simulink model "PPC_P1"  (R2019b)
settings: Solver=ode45  StartTime=0.0  StopTime=50  MaxStep=0.01  RelTol=1e-6
undefined symbols (not defined in the file or in its folder): sigbuilder_block
libraries: slctrlblks x2, simulink x1
settings Model: Creator=Kevin  LastModifiedBy=Kevin

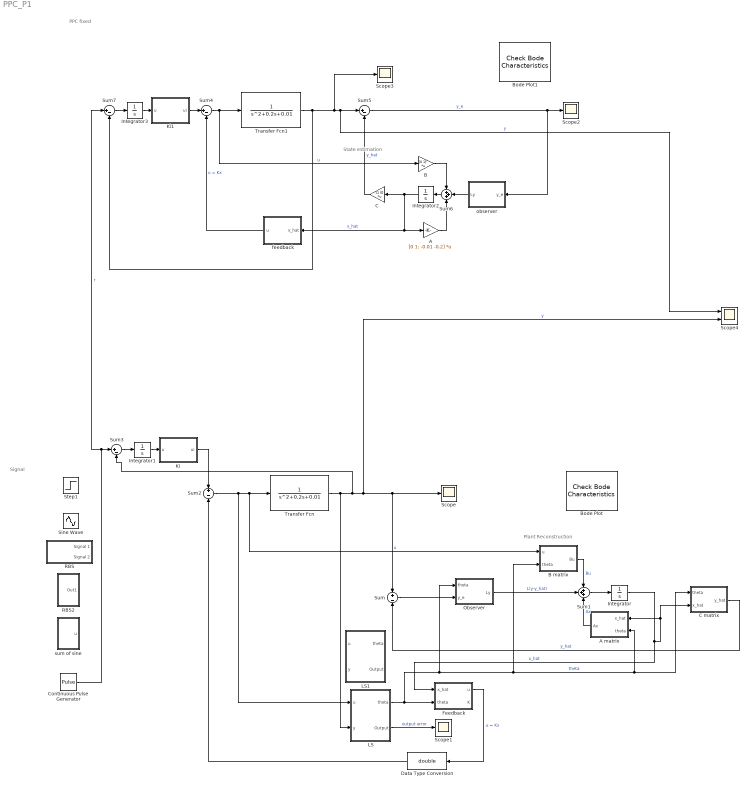
== system PPC_P1 ==
  note: PPC fixed
  note: Plant Reconstruction
  note: Signal
  note: State estimation
  A : Gain  Gain=[0 1; -0.01 -0.2]  Multiplication=Matrix(K*u)
  A matrix : MATLAB Function  TreatAsAtomicUnit=on
  B : Gain  Gain=[0 1]'  Multiplication=Matrix(K*u)
  B matrix : MATLAB Function  TreatAsAtomicUnit=on
  Bode Plot : slctrlblks/Model Verification/Check Bode  Characteristics  InstantiateOnLoad=on  SaveOperatingPoints=off  LinearizationIOs={'/Sum2', 1, 'in', 'off', '';'/Transfer Fcn', 1, 'out', 'on', ''}  LinearizeAt=SnapshotTimes  SnapshotTimes=[0]  TriggerType=rising  SampleTime=auto  RateConversionMethod=zoh  PreWarpFreq=10  UseExactDelayModel=off  UseFullBlockNameLabels=off  UseBusSignalLabels=off  enabled=on  stopWhenAssertionFail=off  export=off  ViewDlgPos=[1921 -319 1920 967.333333333333]  OpenViewOnLoad=off  LaunchViewOnOpen=off  FrequencyUnits=rad/s  MagnitudeUnits=dB  PhaseUnits=deg  TimeUnits=seconds  EnableUpperBound=off  UpperBoundFrequencies=[]  UpperBoundMagnitudes=[]  EnableLowerBound=off  LowerBoundFrequencies=[]  LowerBoundMagnitudes=[]
      settings: SourceProductName=Simulink Control Design
  Bode Plot1 : slctrlblks/Model Verification/Check Bode  Characteristics  InstantiateOnLoad=on  SaveOperatingPoints=off  LinearizationIOs={'/Sum', 1, 'in', 'off', '';'/Transfer Fcn', 1, 'out', 'on', ''}  LinearizeAt=SnapshotTimes  SnapshotTimes=[0]  TriggerType=rising  SampleTime=auto  RateConversionMethod=zoh  PreWarpFreq=10  UseExactDelayModel=off  UseFullBlockNameLabels=off  UseBusSignalLabels=off  enabled=on  stopWhenAssertionFail=off  export=off  ViewDlgPos=[1921 -319 1920 967.333333333333]  OpenViewOnLoad=off  LaunchViewOnOpen=off  FrequencyUnits=rad/s  MagnitudeUnits=dB  PhaseUnits=deg  TimeUnits=seconds  EnableUpperBound=off  UpperBoundFrequencies=[]  UpperBoundMagnitudes=[]  EnableLowerBound=off  LowerBoundFrequencies=[]  LowerBoundMagnitudes=[]
      settings: SourceProductName=Simulink Control Design
  C : Gain  Gain=[1 0]  Multiplication=Matrix(K*u)
  C matrix : MATLAB Function  TreatAsAtomicUnit=on
  Continuous Pulse Generator : DiscretePulseGenerator  PulseType=Time based  Period=1  PulseWidth=50
  Data Type Conversion : DataTypeConversion  OutDataTypeStr=double
  Feedback : MATLAB Function  TreatAsAtomicUnit=on
  Integrator{,1..3} (4 alike) : Integrator
  Ki : MATLAB Function  TreatAsAtomicUnit=on
  Ki1 : MATLAB Function  TreatAsAtomicUnit=on
  LS : Subsystem
  LS1 : Subsystem
  "Observer " : MATLAB Function  TreatAsAtomicUnit=on
  "RBS " : Subsystem  Tag=STV Subsys  LoadFcn=sigbuilder_block('load');  StartFcn=sigbuilder_block('start');  StopFcn=sigbuilder_block('stop');  ClipboardFcn=sigbuilder_block('clipboard');  mask(Sigbuilder block){tuvar=[0:10]}
      mask help: Simulink:masks:SigbuilderBlock_MD
      mask init:
      | if ~strcmp(get_param(bdroot(gcbh),'SimulationStatus'),'stopped') tuvar = sigbuilder_block('maskInit'); end
      settings: CopyFcn=sigbuilder_block('copy');  DeleteFcn=sigbuilder_block('delete');  ModelCloseFcn=sigbuilder_block('modelClose');  PreSaveFcn=sigbuilder_block('preSave');  PauseFcn=sigbuilder_block('pause');  ContinueFcn=sigbuilder_block('continue');  NameChangeFcn=sigbuilder_block('namechange');  OpenFcn=sigbuilder_block('open',[215 62.5 550.5 362.5 ]);  CloseFcn=sigbuilder_block('close');
      mask Display: plot(0, 0, 100, 100,[2, 2, 32, 32, 2], [68, 8, 8, 68, 68],[32, 2], [38, 38], [32, 19, 2],[53, 60, 44], [32, 17, 17, 2],[16, 16, 31, 31]);txt = getActiveGroup(gcbh);text(2, 100, txt,'verticalAlignment', 'top');
  RBS2 : Subsystem
  Scope{,1..3} (4 alike) : Scope
  Scope4 : Scope  NumInputPorts=2
  Sine Wave : Sin  Frequency=0.1  SampleTime=0
  Step1 : Step  SampleTime=0
  Sum : Sum  Inputs=+-
  Sum1 : Sum  Inputs=+++
  Sum2 : Sum  Inputs=+-
  Sum{3..5,7} (4 alike) : Sum  Inputs=|+-
  Sum6 : Sum  Inputs=+++
  Transfer Fcn : TransferFcn  Denominator=[1 ,0.2 ,0.01]
  Transfer Fcn1 : TransferFcn  Denominator=[1 ,0.2 ,0.01]
  feedback : MATLAB Function  TreatAsAtomicUnit=on
  "observer " : MATLAB Function  TreatAsAtomicUnit=on
  sum of sine : Subsystem
  wires:
  Transfer Fcn/1 -> LS/2(y), Sum3/2, Scope4/2, Scope/1, Sum/1  "y"
  Sum2/1 -> LS/1("u "), B matrix/1(u), Transfer Fcn/1  "u"
  LS/1(theta) -> C matrix/1(theta), A matrix/2(theta), B matrix/2(theta), "Observer "/1(theta), Feedback/2(theta)  "theta"
  Sum/1 -> "Observer "/2(y_e)
  Sum1/1 -> Integrator/1
  Integrator/1 -> C matrix/2(x_hat), A matrix/1(x_hat), Feedback/1(x_hat)  "x_hat"
  A matrix/1(Ax) -> Sum1/3  "Ax"
  "Observer "/1(Ly) -> Sum1/2  "L(y-y_hat)"
  C matrix/1(y_hat) -> Sum/2  "y_hat"
  Feedback/1(u) -> Data Type Conversion/1  "u = Kx"
  B matrix/1(Bu) -> Sum1/1  "Bu"
  LS/2(Output) -> Scope1/1  "output error"
  Data Type Conversion/1 -> Sum2/2
  Integrator1/1 -> Ki/1(u)
  Sum3/1 -> Integrator1/1
  Ki/1(ui) -> Sum2/1
  Sum6/1 -> Integrator2/1
  B/1 -> Sum6/1
  Ki1/1(ui) -> Sum4/1
  Transfer Fcn1/1 -> Scope3/1, Scope4/1, Sum5/1, Sum7/2  "y"
  Sum7/1 -> Integrator3/1
  Integrator3/1 -> Ki1/1(u)
  Sum5/1 -> "observer "/1(y_e), Scope2/1  "y_e"
  Sum4/1 -> B/1, Transfer Fcn1/1  "u"
  Integrator2/1 -> C/1, feedback/1(x_hat), A/1  "x_hat"
  Continuous Pulse Generator/1 -> Sum3/1, Sum7/1  "r"
  "observer "/1(Ly) -> Sum6/2
  A/1 -> Sum6/3
  feedback/1(u) -> Sum4/2  "u = Kx"
  C/1 -> Sum5/2  "y_hat"

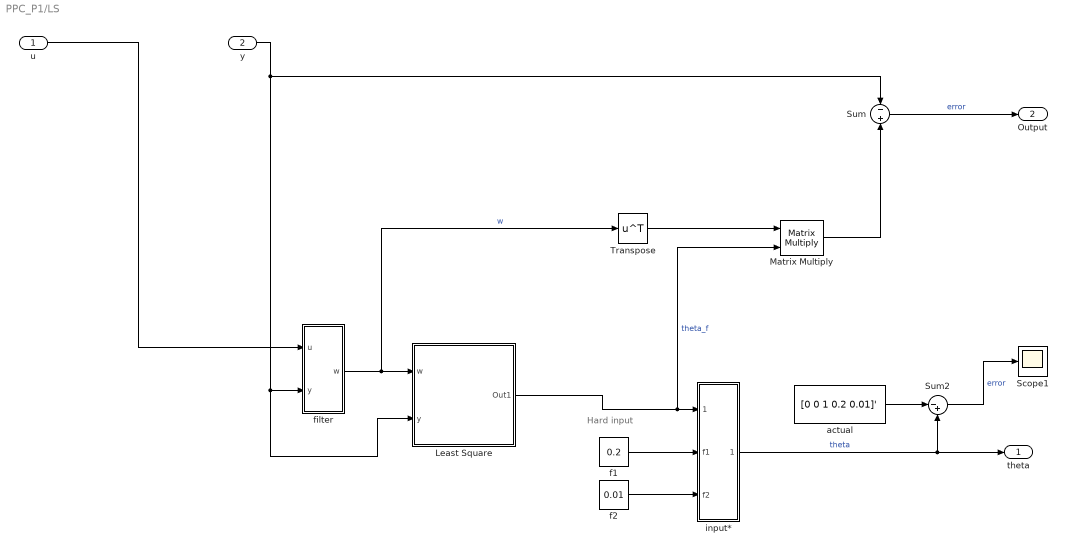
== system PPC_P1/LS ==
  note: Hard input
  "u " : Inport
  y : Inport  Port=2
  Least Square : Subsystem
  Matrix Multiply : Product  Multiplication=Matrix(*)
  Scope1 : Scope
  Sum : Sum  Inputs=-+
  Sum2 : Sum  Inputs=|-+
  Transpose : Math  Operator=transpose  SignedPower=off  SaturateOnIntegerOverflow=on
  actual : Constant  Value=[0 0 1 0.2 0.01]'
  f1 : Constant  Value=0.2
  f2 : Constant  Value=0.01
  "filter " : Subsystem
  input* : Subsystem
  theta : Outport
  Output : Outport  Port=2
  wires:
  y/1 -> Sum/1, Least Square/2(y), "filter "/2("y ")
  Sum2/1 -> Scope1/1  "error"
  f2/1 -> input*/3(f2)
  actual/1 -> Sum2/1
  "u "/1 -> "filter "/1("u ")
  f1/1 -> input*/2(f1)
  Least Square/1(Out1) -> Matrix Multiply/2, input*/1(theta_f)  "theta_f"
  input*/1(Out1) -> Sum2/2, theta/1  "theta"
  "filter "/1(w) -> Transpose/1, Least Square/1(w)  "w"
  Transpose/1 -> Matrix Multiply/1
  Matrix Multiply/1 -> Sum/2
  Sum/1 -> Output/1  "error"

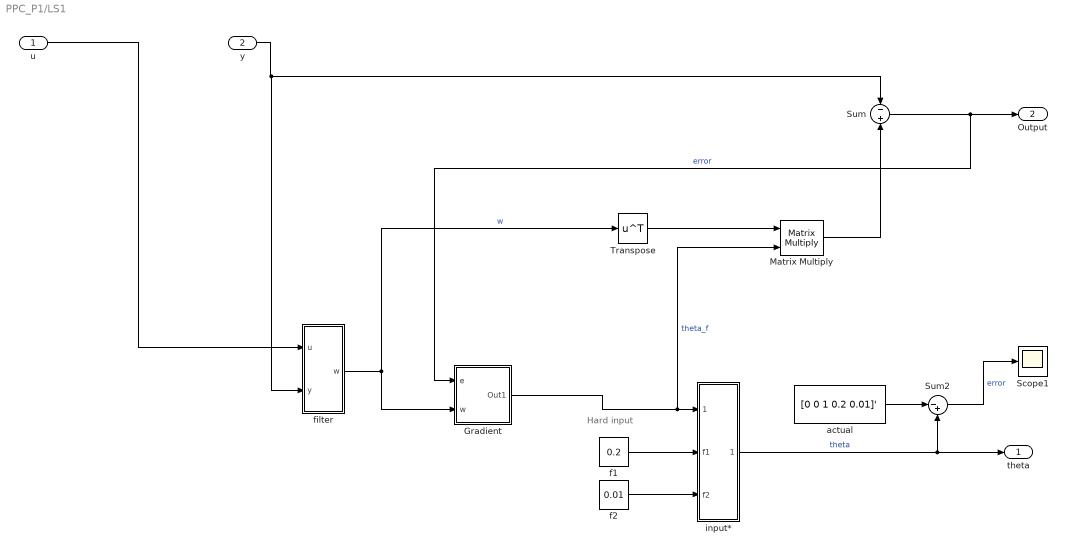
== system PPC_P1/LS1 ==
  note: Hard input
  "u " : Inport
  y : Inport  Port=2
  Gradient : Subsystem
  Matrix Multiply : Product  Multiplication=Matrix(*)
  Scope1 : Scope
  Sum : Sum  Inputs=-+
  Sum2 : Sum  Inputs=|-+
  Transpose : Math  Operator=transpose  SignedPower=off  SaturateOnIntegerOverflow=on
  actual : Constant  Value=[0 0 1 0.2 0.01]'
  f1 : Constant  Value=0.2
  f2 : Constant  Value=0.01
  "filter " : Subsystem
  input* : Subsystem
  theta : Outport
  Output : Outport  Port=2
  wires:
  y/1 -> "filter "/2("y "), Sum/1
  Sum2/1 -> Scope1/1  "error"
  f2/1 -> input*/3(f2)
  actual/1 -> Sum2/1
  "u "/1 -> "filter "/1("u ")
  f1/1 -> input*/2(f1)
  Gradient/1(Out1) -> Matrix Multiply/2, input*/1(theta_f)  "theta_f"
  input*/1(Out1) -> Sum2/2, theta/1  "theta"
  "filter "/1(w) -> Gradient/2(w), Transpose/1  "w"
  Transpose/1 -> Matrix Multiply/1
  Matrix Multiply/1 -> Sum/2
  Sum/1 -> Gradient/1(e), Output/1  "error"

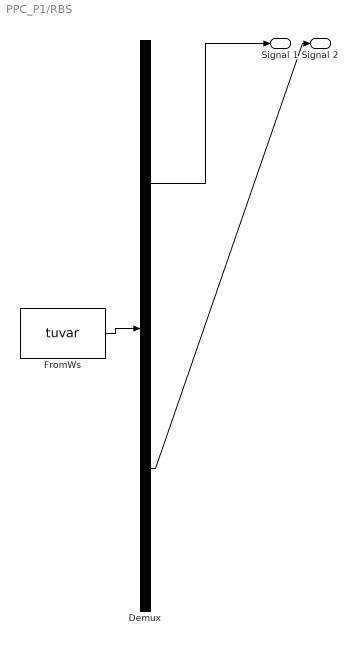
== system PPC_P1/RBS  ==
  Demux : Demux  Tag=STV Demux  Outputs=2
  FromWs : FromWorkspace  Tag=STV FromWs  VariableName=tuvar  SampleTime=0
      SigBuilderData=|
      | common.afterFinalStr = 'Extrapolate'
      | common.sampleTime = 0
      | dataSet.timeRange = [0 10]
      | dataSet.name = 'Group 1'
      | sbobj.Groups.Name = 'Group 1'
      | sbobj.Groups.Signals(1).Name = 'Signal 1'
      | sbobj.Groups.Signals(1).XData = [0 4 4 6 6 10]
      | sbobj.Groups.Signals(1).YData = [0 0 1 1 0 0]
      | sbobj.Groups.Signals(2).Name = 'Signal 2'
      | sbobj.Groups.Signals(2).XData = [0 0.2 0.2 0.3 0.3 0.5 0.5 0.7 0.7 1 1 1.1 1.1 1.3 1.3 1.4 1.4 1.5 1.5 1.7 1.7 2.1 2.1 2.2 2.2 2.7 2.7 2.8 2.8 2.9 2.9 3 3 3.1 3.1 3.5 3.5 3.7 3.7 3.8 3.8 3.9 3.9 4.2 4.2 4.4 4.4 4.7 4.7 5 5 5.1 5.1 5.3 5.3 5.6 5.6 5.7 5.7 5.8 5.8 5.9 5.9 6 6 6.1 6.1 6.2 6.2 6.7 6.7 7 7 7.1 7.1 7.2 7.2 7.3 7.3 7.4 7.4 7.5 7.5 7.8 7.8 7.9 7.9 8.1 8.1 8.5 8.5 8.6 8.6 8.8 8.8 8.9 8.9 9 9 9.2 9.2 9.5 9.5 9.6 9.6 9.7 9.7 10]
      | sbobj.Groups.Signals(2).YData = [1 1 0 0 1 1 0 0 1 1 0 0 1 1 0 0 1 1 0 0 1 1 0 0 1 1 0 0 1 1 0 0 1 1 0 0 1 1 0 0 1 1 0 0 1 1 0 0 1 1 0 0 1 1 0 0 1 1 0 0 1 1 0 0 1 1 0 0 1 1 0 0 1 1 0 0 1 1 0 0 1 1 0 0 1 1 0 0 1 1 0 0 1 1 0 0 1 1 0 0 1 1 0 0 1 1 0 0]
  Signal 1 : Outport  Tag=STV Outport
  Signal 2 : Outport  Tag=STV Outport  Port=2
  wires:
  Demux/1 -> Signal 1/1
  FromWs/1 -> Demux/1
  Demux/2 -> Signal 2/1

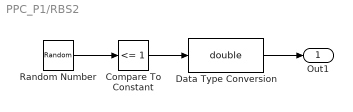
== system PPC_P1/RBS2 ==
  Compare To Constant : simulink/Logic and Bit Operations/Compare To Constant  relop=<=  const=1  OutDataTypeStr=boolean
  Data Type Conversion : DataTypeConversion  OutDataTypeStr=double
  Random Number : RandomNumber  Mean=1  SampleTime=10
  Out1 : Outport
  wires:
  Random Number/1 -> Compare To Constant/1
  Compare To Constant/1 -> Data Type Conversion/1
  Data Type Conversion/1 -> Out1/1

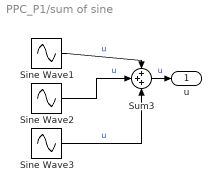
== system PPC_P1/sum of sine ==
  Sine Wave1 : Sin  Frequency=0.1  Phase=0.1  SampleTime=0
  Sine Wave2 : Sin  SampleTime=0
  Sine Wave3 : Sin  Frequency=2  SampleTime=0
  Sum3 : Sum  Inputs=+++
  u : Outport
  wires:
  Sine Wave3/1 -> Sum3/3  "u"
  Sine Wave1/1 -> Sum3/1  "u"
  Sum3/1 -> u/1  "u"
  Sine Wave2/1 -> Sum3/2  "u"

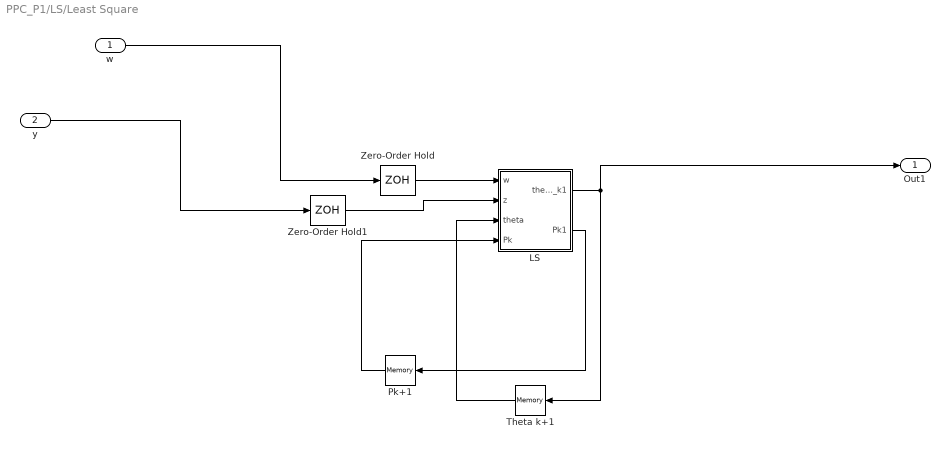
== system PPC_P1/LS/Least Square ==
  w : Inport
  y : Inport  Port=2
  LS : MATLAB Function  TreatAsAtomicUnit=on
  Pk+1 : Memory  InitialCondition=(10^5)*eye(5)  InheritSampleTime=on
  Theta k+1 : Memory  InitialCondition=[0.1 0 1.1 0.1 0.1]'  InheritSampleTime=on
  Zero-Order Hold : ZeroOrderHold  SampleTime=0.01
  Zero-Order Hold1 : ZeroOrderHold  SampleTime=0.01
  Out1 : Outport
  wires:
  Zero-Order Hold/1 -> LS/1(w)
  Pk+1/1 -> LS/4(Pk)
  Zero-Order Hold1/1 -> LS/2(z)
  LS/1(theta_k1) -> Out1/1, Theta k+1/1
  y/1 -> Zero-Order Hold1/1
  LS/2(Pk1) -> Pk+1/1
  Theta k+1/1 -> LS/3(theta)
  w/1 -> Zero-Order Hold/1

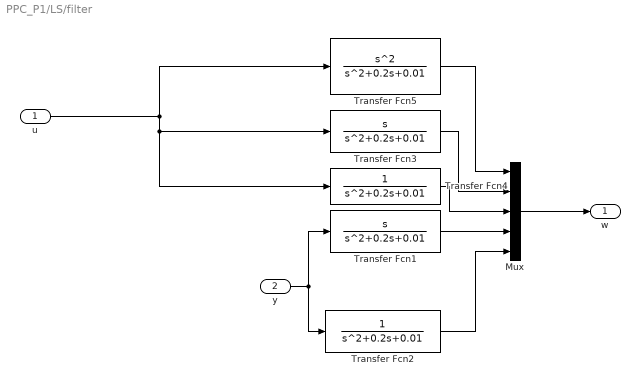
== system PPC_P1/LS/filter  ==
  "u " : Inport
  "y " : Inport  Port=2
  Mux : Mux  Inputs=5
  Transfer Fcn1 : TransferFcn  Numerator=[1 0]  Denominator=[1 0.2 0.01]
  Transfer Fcn2 : TransferFcn  Denominator=[1 0.2 0.01]
  Transfer Fcn3 : TransferFcn  Numerator=[1 0]  Denominator=[1 0.2 0.01]
  Transfer Fcn4 : TransferFcn  Denominator=[1 0.2 0.01]
  Transfer Fcn5 : TransferFcn  Numerator=[1 0 0]  Denominator=[1 0.2 0.01]
  w : Outport
  wires:
  Transfer Fcn1/1 -> Mux/4
  "u "/1 -> Transfer Fcn4/1, Transfer Fcn3/1, Transfer Fcn5/1
  Mux/1 -> w/1
  "y "/1 -> Transfer Fcn1/1, Transfer Fcn2/1
  Transfer Fcn2/1 -> Mux/5
  Transfer Fcn5/1 -> Mux/1
  Transfer Fcn3/1 -> Mux/2
  Transfer Fcn4/1 -> Mux/3

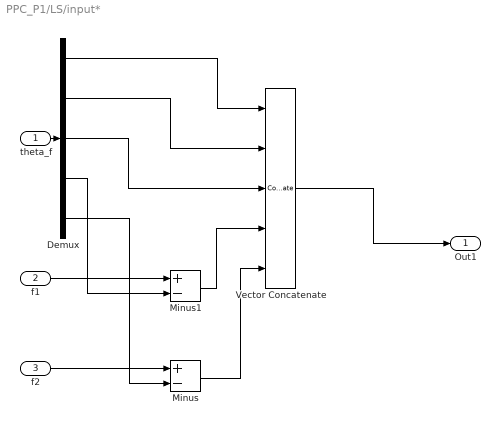
== system PPC_P1/LS/input* ==
  theta_f : Inport
  f1 : Inport  Port=2
  f2 : Inport  Port=3
  Demux : Demux  Outputs=5
  Minus : Sum  Inputs=+-
  Minus1 : Sum  Inputs=+-
  Vector Concatenate : Concatenate  NumInputs=5
  Out1 : Outport
  wires:
  Vector Concatenate/1 -> Out1/1
  Minus1/1 -> Vector Concatenate/4
  Minus/1 -> Vector Concatenate/5
  Demux/1 -> Vector Concatenate/1
  Demux/4 -> Minus1/2
  Demux/3 -> Vector Concatenate/3
  Demux/5 -> Minus/2
  f2/1 -> Minus/1
  Demux/2 -> Vector Concatenate/2
  f1/1 -> Minus1/1
  theta_f/1 -> Demux/1

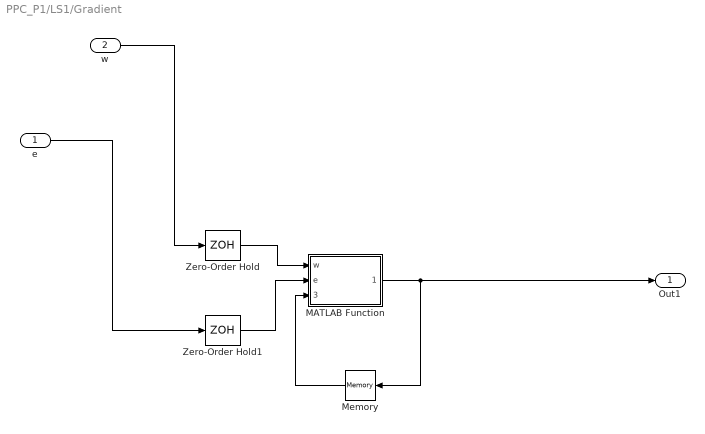
== system PPC_P1/LS1/Gradient ==
  e : Inport
  w : Inport  Port=2
  MATLAB Function : MATLAB Function  TreatAsAtomicUnit=on
  Memory : Memory  InitialCondition=[0 0 0.9 0.000001 0.0000001]'  InheritSampleTime=on
  Zero-Order Hold : ZeroOrderHold  SampleTime=0.01
  Zero-Order Hold1 : ZeroOrderHold  SampleTime=0.01
  Out1 : Outport
  wires:
  MATLAB Function/1(theta_k1) -> Memory/1, Out1/1
  Zero-Order Hold/1 -> MATLAB Function/1(w)
  w/1 -> Zero-Order Hold/1
  Zero-Order Hold1/1 -> MATLAB Function/2(e)
  e/1 -> Zero-Order Hold1/1
  Memory/1 -> MATLAB Function/3(theta_1)

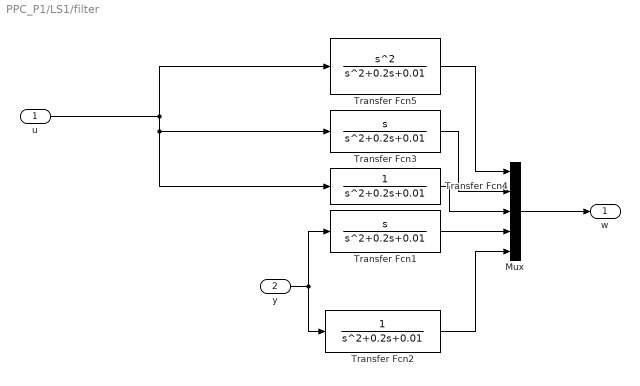
== system PPC_P1/LS1/filter  ==
  "u " : Inport
  "y " : Inport  Port=2
  Mux : Mux  Inputs=5
  Transfer Fcn1 : TransferFcn  Numerator=[1 0]  Denominator=[1 0.2 0.01]
  Transfer Fcn2 : TransferFcn  Denominator=[1 0.2 0.01]
  Transfer Fcn3 : TransferFcn  Numerator=[1 0]  Denominator=[1 0.2 0.01]
  Transfer Fcn4 : TransferFcn  Denominator=[1 0.2 0.01]
  Transfer Fcn5 : TransferFcn  Numerator=[1 0 0]  Denominator=[1 0.2 0.01]
  w : Outport
  wires:
  Transfer Fcn1/1 -> Mux/4
  "u "/1 -> Transfer Fcn4/1, Transfer Fcn3/1, Transfer Fcn5/1
  Mux/1 -> w/1
  "y "/1 -> Transfer Fcn1/1, Transfer Fcn2/1
  Transfer Fcn2/1 -> Mux/5
  Transfer Fcn5/1 -> Mux/1
  Transfer Fcn3/1 -> Mux/2
  Transfer Fcn4/1 -> Mux/3

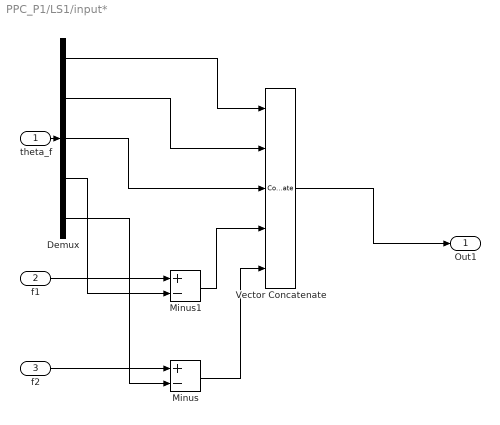
== system PPC_P1/LS1/input* ==
  theta_f : Inport
  f1 : Inport  Port=2
  f2 : Inport  Port=3
  Demux : Demux  Outputs=5
  Minus : Sum  Inputs=+-
  Minus1 : Sum  Inputs=+-
  Vector Concatenate : Concatenate  NumInputs=5
  Out1 : Outport
  wires:
  Vector Concatenate/1 -> Out1/1
  Minus1/1 -> Vector Concatenate/4
  Minus/1 -> Vector Concatenate/5
  Demux/1 -> Vector Concatenate/1
  Demux/4 -> Minus1/2
  Demux/3 -> Vector Concatenate/3
  Demux/5 -> Minus/2
  f2/1 -> Minus/1
  Demux/2 -> Vector Concatenate/2
  f1/1 -> Minus1/1
  theta_f/1 -> Demux/1

== matlab function PPC_P1/LS/Least Square/LS ==
  data: w input; z input; theta input; Pk input; theta_k1 output; Pk1 output
function [ theta_k1,Pk1] = fcn(w, z, theta, Pk)
alpha = 1; %standard
gamma = 1/alpha;
%e = 10^-4;
%Q = e*eye(5);
%Pk = eye(5);

%initial values
%ro = 10^5;
%P1 = ro*eye(5);
%theta1 = [0 0 1 0.2 0.01]';
%Calculations

theta_k1 = theta - (gamma*Pk*w*(w'*theta-z))/ (1+gamma*w'*Pk*w);
Pk1 = (1/alpha)*Pk - ((gamma^2*Pk*w*w'*Pk)/(1+gamma*w'*Pk*w));

== matlab function PPC_P1/Ki ==
  data: u input; ui output
function ui = fcn(u)
 coder.extrinsic("ss","place","matsplit",'ctrb');
% [b2, b1, b0, a1, a0] = matsplit(theta);
ui = 0;
A = [0 1; -0.01 -0.2];
B = [0 1]';
C = [1 0];

o = [0 0]';
A1 = [A o;C 0];
B1 = [B;0];
p = [-30+0.69805i -30-0.69805i -50];
K1 = place(A1,B1,p);
Ki = [K1(3)];
ui = Ki*u;

== matlab function PPC_P1/LS1/Gradient/MATLAB Function ==
  data: w input; theta_k1 output; e input; theta_1 input
function theta_k1 = fcn(w, e, theta_1)
%gamma = 0.000001;
theta_k1 = [0 0 0 0 0]';
theta_dot = [0 0 0 0 0]';

alpha = 0.000001;
dt = 0.01;
I = eye(5);
gamma = alpha*I;
theta_dot = -gamma*w*e;
theta_k1 = theta_1 + theta_dot*dt;

== matlab function PPC_P1/Feedback ==
  data: x_hat input; theta input; u output; K output
function [u,K] = fcn(x_hat, theta)
 coder.extrinsic("ss","place","matsplit",'ctrb');
% [b2, b1, b0, a1, a0] = matsplit(theta);
K = [0 0];
u = 0;
A = [0 1; -theta(5) -theta(4)];
B = [0 1]';
C = [theta(3) theta(2)];
% D = 0;
% %sys = ss(A,B,C,D);
% p = [-.1+0.69805i -.1-0.69805i];
% K = place(A,B,p);

% a0 = theta(5); a1 = theta(4); %values of A in CCF
% p1 = -1; p2 = -1; % desired pole values
% alpha = [-(p1+p2) p1*p2];
% P = ctrb(A,B);
% Pccf1 = [a1 1; 1 0];
% 
% K = [alpha(2)-a0 alpha(1)-a1]*inv(P*Pccf1);
o = [0 0]';
A1 = [A o;C 0];
B1 = [B;0];
p = [-30+0.69805i -30-0.69805i -50];
K1 = place(A1,B1,p);
K = [K1(1) K1(2)];
u = K*x_hat;

== matlab function PPC_P1/Observer  ==
  data: theta input; y_e input; Ly output
function Ly = fcn(theta, y_e)
 coder.extrinsic('ss','place','pole','matsplit','complex','real','imag','ctrb');
 Ly = [0 0];
% %place pole 10 times to the left from the actual plant
% %[b2, b1, b0, a1, a0] = matsplit(theta);
A = [0 1; -theta(5) -theta(4)];
B = [0 1]';
C = [theta(3) theta(2)];
%sys = ss(A,B,C,0);
%p = pole(sys);
%p_des = [complex(10*real(p(1)),imag(p(1))) complex(10*real(p(2)),imag(p(2)))];
% p1 = complex(10*real(p(1)),imag(p(1)));
% p2 = complex(10*real(p(2)),imag(p(2)));
% p_des = [-10+i -10-i];
% L = place(A,C,p_des);
% p1 = real(p(1))*10;
% p2 = real(p(2))*10;
a0 = theta(5);
a1 = theta(4);
P = ctrb(A,B);
Pccf1 = [a1 1; 1 0];
 p1 = -10; p2 = -10; 
 alpha = [-(p1+p2) p1*p2];

 L = [alpha(2)-a0 alpha(1)-a1]*inv(P*Pccf1);
Ly = L*y_e;

== matlab function PPC_P1/Ki1 ==
  data: u input; ui output
function ui = fcn(u)
 coder.extrinsic("ss","place","matsplit",'ctrb');
% [b2, b1, b0, a1, a0] = matsplit(theta);
ui = 0;
A = [0 1; -0.01 -0.2];
B = [0 1]';
C = [1 0];

o = [0 0]';
A1 = [A o;C 0];
B1 = [B;0];
p = [-30+0.69805i -30-0.69805i -50];
K1 = place(A1,B1,p);
Ki = [K1(3)];
ui = Ki*u;

== matlab function PPC_P1/C matrix ==
  data: theta input; x_hat input; y_hat output
function y_hat = fcn(theta, x_hat)
%coder.extrinsic("matsplit");
%[b2, b1, b0, a1, a0] = matsplit(theta);
%C = [b0 b1];
C = [theta(3) theta(2)];
y_hat = C*x_hat;

== matlab function PPC_P1/A matrix ==
  data: x_hat input; Ax output; theta input
function Ax = fcn(x_hat, theta)
%coder.extrinsic("matsplit");
%[b2, b1, b0, a1, a0] = matsplit(theta);
A = [0 1; -theta(5) -theta(4)];

Ax = A*x_hat;

== matlab function PPC_P1/B matrix ==
  data: u input; Bu output; theta input
function Bu = fcn(u, theta)
%coder.extrinsic("matsplit");
%[b2, b1, b0, a1, a0] = matsplit(theta);
B = [0 1]';
Bu = B*u;

== matlab function PPC_P1/feedback ==
  data: x_hat input; u output
function u = fcn(x_hat)
 coder.extrinsic("ss","place","matsplit",'ctrb');
% [b2, b1, b0, a1, a0] = matsplit(theta);
K = [0 0];
u = 0;
A = [0 1; -0.01 -0.2];
B = [0 1]';
C = [1 0];

%servomechanism
o = [0 0]';
A1 = [A o;C 0];
B1 = [B;0];
p = [-30+0.69805i -30-0.69805i -50]; %let third pole be less affective
K1 = place(A1,B1,p);
K = [K1(1) K1(2)];
u = K*x_hat;

== matlab function PPC_P1/observer  ==
  data: y_e input; Ly output
function Ly  = fcn(y_e)
coder.extrinsic("ss","place","matsplit",'ctrb');
Ly = [0 0];
A = [0 1; -0.01 -0.2];
B = [0 1]';
C = [1 0];

%observer design
a0 = 0.01;
a1 = 0.2;
P = ctrb(A,B);
Pccf1 = [a1 1; 1 0];
p1 = -10; p2 = -10; 
alpha = [-(p1+p2) p1*p2];
L = [alpha(2)-a0 alpha(1)-a1]*inv(P*Pccf1);
Ly = L*y_e;
